simulink library "csc_lac_landing_acceleration_command_lib"  (R2015b)
settings: Solver=ode45  StartTime=0.0  StopTime=10.0  RelTol=1e-3
values from neighbouring files (symbols this model uses):
  lac_accel_available_init = 1    [csc_lac_landing_acceleration_command_init.m]
  lac_bias_on_perfect = -1.0    (= -1)    [csc_lac_landing_acceleration_command_init.m]
  lac_coarse_acs_thrust_available = psp_coarse_acs_thrust*4    [csc_lac_landing_acceleration_command_prep.m]
  lac_main_biprop_thrust_available = psp_main_biprop_thrust    [csc_lac_landing_acceleration_command_prep.m]
  lac_monoprop_coarse_transition_alt = 1e6    (= 1000000)    [csc_lac_landing_acceleration_command_init.m]
  lac_perfect_vel_nav = 1    [csc_lac_landing_acceleration_command_init.m]
undefined symbols (not defined in the file or in its folder): csc_gdn_dt
libraries: util_common_lib x4, simulink x1, util_info_lib x1, csc_ltg_landing_terminal_guidance_lib x1, csu_lat_landing_approach_targeting_lib x1, csu_lpc_landing_pre_coast_lib x1
settings Model: Creator=escrane  LastModifiedBy=jkaidy
settings DataIOCC: SaveFormat=Array
settings DebuggingCC: UnderspecifiedInitializationDetection=Classic  MergeDetectMultiDrivingBlocksExec=none  SolverPrmCheckMsg=warning
settings HardwareCC: ProdBitPerPointer=32  ProdLargestAtomicFloat=None  ProdIntDivRoundTo=Undefined  ProdEndianess=Unspecified  ProdWordSize=32  ProdHWDeviceType=32-bit Generic
settings GRTTargetCC: GeneratePreprocessorConditionals=Disable all
settings ConfigComp: CovModelRefEnable=Off  CovSFcnEnable=off

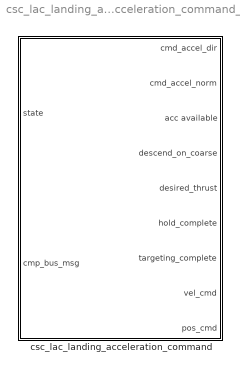
== system csc_lac_landing_acceleration_command_lib ==
  csc_lac_landing_acceleration_command : Subsystem

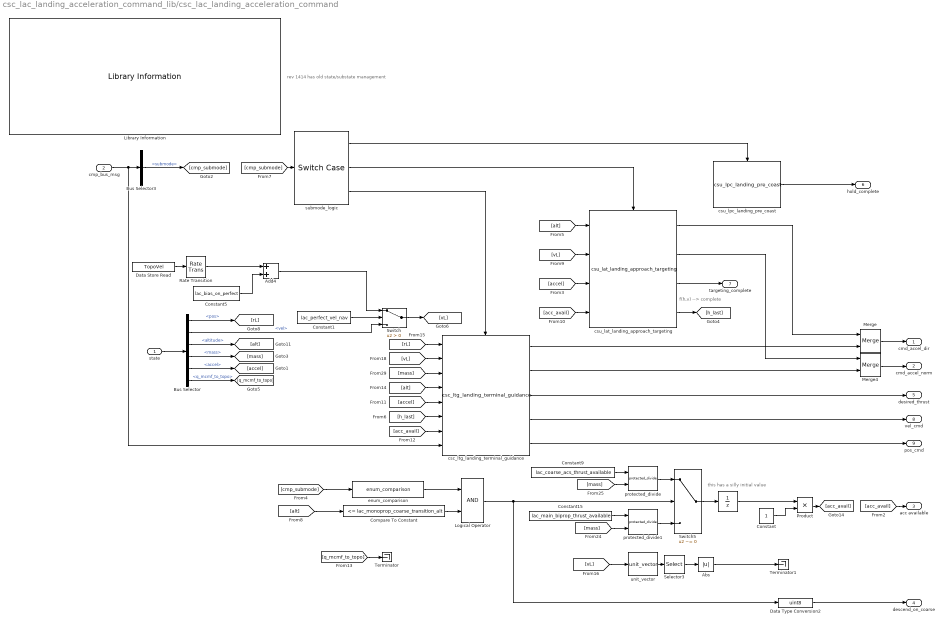
== system csc_lac_landing_acceleration_command_lib/csc_lac_landing_acceleration_command ==
  note: this has a silly initial value
  note: f(h,v) --> complete
  note: rev 1414 has old state/substate management
  state : Inport
  cmp_bus_msg : Inport  Port=2
  " " : UnitDelay  InitialCondition=lac_accel_available_init  SampleTime=csc_gdn_dt
  Abs : Abs
  Add4 : Sum
  Bus Selector : BusSelector  OutputSignals=pos,vel,altitude,mass,accel,q_mcmf_to_topo
  Bus Selector3 : BusSelector  OutputSignals=submode
  Compare To Constant : simulink/Logic and Bit Operations/Compare To Constant  relop=<=  const=lac_monoprop_coarse_transition_alt  OutDataTypeStr=boolean
  Constant : Constant
  Constant1 : Constant  Value=lac_perfect_vel_nav
  Constant15 : Constant  Value=lac_main_biprop_thrust_available
  Constant5 : Constant  Value=lac_bias_on_perfect
  Constant9 : Constant  Value=lac_coarse_acs_thrust_available
  Data Store Read : DataStoreRead  DataStoreName=TopoVel
  Data Type Conversion2 : DataTypeConversion  OutDataTypeStr=uint8
  Library Information : util_info_lib/Library Information  owner='NONE'
  Logical Operator : Logic  AllPortsSameDT=off  OutDataTypeStr=boolean
  Merge : Merge  InitialOutput=[-1 0 0]'
  Merge4 : Merge  InitialOutput=0
  Product : Product
  Rate Transition : RateTransition
  Selector3 : Selector  InputPortWidth=3  IndexOptions=Index vector (dialog)  Indices=[3]  OutputSizes=1
  Switch : Switch  Criteria=u2 > Threshold
  Switch5 : Switch  Criteria=u2 ~= 0
  Terminator : Terminator
  Terminator1 : Terminator
  csc_ltg_landing_terminal_guidance : csc_ltg_landing_terminal_guidance_lib/csc_ltg_landing_terminal_guidance
  csu_lat_landing_approach_targeting : csu_lat_landing_approach_targeting_lib/csu_lat_landing_approach_targeting
  csu_lpc_landing_pre_coast : csu_lpc_landing_pre_coast_lib/csu_lpc_landing_pre_coast
  enum_comparison : util_common_lib/enum_comparison  comparison_type===
  protected_divide : util_common_lib/protected_divide  fault_value=0  tolerance=eps
  protected_divide1 : util_common_lib/protected_divide  fault_value=0  tolerance=eps
  submode_logic : SwitchCase  CaseConditions={uint8(enum_submode.landing_hold), uint8(enum_submode.landing_targeting), uint8(enum_submode.landing_terminal)}  ShowDefaultCase=off
  unit_vector : util_common_lib/unit_vector  SystemSampleTime=-1
  cmd_accel_dir : Outport
  cmd_accel_norm : Outport  Port=2
  acc available : Outport  Port=3
  descend_on_coarse : Outport  Port=4  InitialOutput=1
  desired_thrust : Outport  Port=5
  hold_complete : Outport  Port=6
  targeting_complete : Outport  Port=7
  vel_cmd : Outport  Port=8
  pos_cmd : Outport  Port=9
  wires:
  Bus Selector/6 -> [q_mcmf_to_topo]  "<q_mcmf_to_topo>"
  csc_ltg_landing_terminal_guidance/5 -> pos_cmd/1
  csc_ltg_landing_terminal_guidance/4 -> vel_cmd/1
  Bus Selector/1 -> [rL]  "<pos>"
  submode_logic/3 -> csc_ltg_landing_terminal_guidance/Action
  Constant15/1 -> protected_divide1/1
  Constant9/1 -> protected_divide/1
  csu_lat_landing_approach_targeting/3 -> targeting_complete/1
  Bus Selector/4 -> [mass]  "<mass>"
  [cmp_submode] -> submode_logic/1
  csc_ltg_landing_terminal_guidance/1 -> Merge/2
  csc_ltg_landing_terminal_guidance/2 -> Merge4/2
  Bus Selector3/1 -> [cmp_submode]  "<submode>"
  csu_lpc_landing_pre_coast/1 -> hold_complete/1
  Compare To Constant/1 -> Logical Operator/2
  enum_comparison/1 -> Logical Operator/1
  [cmp_submode] -> enum_comparison/1
  submode_logic/2 -> csu_lat_landing_approach_targeting/Action
  submode_logic/1 -> csu_lpc_landing_pre_coast/Action
  [accel] -> csc_ltg_landing_terminal_guidance/5
  Bus Selector/5 -> [accel]  "<accel>"
  [vL] -> csu_lat_landing_approach_targeting/2
  [alt] -> csu_lat_landing_approach_targeting/1
  state/1 -> Bus Selector/1
  [rL] -> csc_ltg_landing_terminal_guidance/1
  [vL] -> csc_ltg_landing_terminal_guidance/2
  Bus Selector/3 -> [alt]  "<altitude>"
  Merge/1 -> cmd_accel_dir/1
  Merge4/1 -> cmd_accel_norm/1
  csu_lat_landing_approach_targeting/1 -> Merge/1
  csu_lat_landing_approach_targeting/2 -> Merge4/1
  [acc_avail] -> acc available/1
  Bus Selector/2 -> Switch/3  "<vel>"
  Logical Operator/1 -> Switch5/2, Data Type Conversion2/1
  Switch5/1 -> " "/1
  csc_ltg_landing_terminal_guidance/3 -> desired_thrust/1
  [mass] -> protected_divide/2
  [mass] -> protected_divide1/2
  protected_divide1/1 -> Switch5/3
  protected_divide/1 -> Switch5/1
  Data Type Conversion2/1 -> descend_on_coarse/1
  [mass] -> csc_ltg_landing_terminal_guidance/3
  cmp_bus_msg/1 -> csc_ltg_landing_terminal_guidance/8, Bus Selector3/1
  [alt] -> csc_ltg_landing_terminal_guidance/4
  [alt] -> Compare To Constant/1
  unit_vector/1 -> Selector3/1
  Selector3/1 -> Abs/1
  " "/1 -> Product/1
  Product/1 -> [acc_avail]
  Abs/1 -> Terminator1/1
  [acc_avail] -> csu_lat_landing_approach_targeting/4
  [accel] -> csu_lat_landing_approach_targeting/3
  [h_last] -> csc_ltg_landing_terminal_guidance/6
  [acc_avail] -> csc_ltg_landing_terminal_guidance/7
  csu_lat_landing_approach_targeting/4 -> [h_last]
  [q_mcmf_to_topo] -> Terminator/1
  [vL] -> unit_vector/1
  Constant/1 -> Product/2
  Switch/1 -> [vL]
  Constant1/1 -> Switch/2
  Data Store Read/1 -> Rate Transition/1
  Constant5/1 -> Add4/2
  Rate Transition/1 -> Add4/1
  Add4/1 -> Switch/1
